simulink model "link1"  (R2016b)
settings: Solver=VariableStepAuto  StartTime=0.0  StopTime=10.0  RelTol=1e-3
settings Model: Creator=gz199  LastModifiedBy=gz199

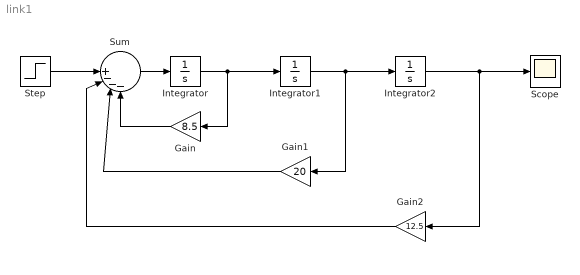
== system link1 ==
  Gain : Gain  Gain=8.5
  Gain1 : Gain  Gain=20
  Gain2 : Gain  Gain=12.5
  Integrator : Integrator
  Integrator1 : Integrator
  Integrator2 : Integrator
  Scope : Scope
  Step : Step  SampleTime=0
  Sum : Sum  Inputs=|||+---
  wires:
  Step/1 -> Sum/1
  Sum/1 -> Integrator/1
  Gain2/1 -> Sum/2
  Gain1/1 -> Sum/3
  Gain/1 -> Sum/4
  Integrator/1 -> Gain/1, Integrator1/1
  Integrator1/1 -> Gain1/1, Integrator2/1
  Integrator2/1 -> Gain2/1, Scope/1
